simulink model "zhuangtaiguanceqi"  (R2022b)
settings: Solver=VariableStepAuto  StartTime=0.0  StopTime=100  RelTol=1e-3
settings Model: Creator=HONOR  LastModifiedBy=acer
settings DebuggingCC: UnconnectedInputMsg=warning  UnconnectedOutputMsg=warning  UnconnectedLineMsg=warning
settings ModelReferenceCC: EnableRefExpFcnMdlSchedulingChecks=on
settings RTWCC: DLArmComputeVersion=19.05

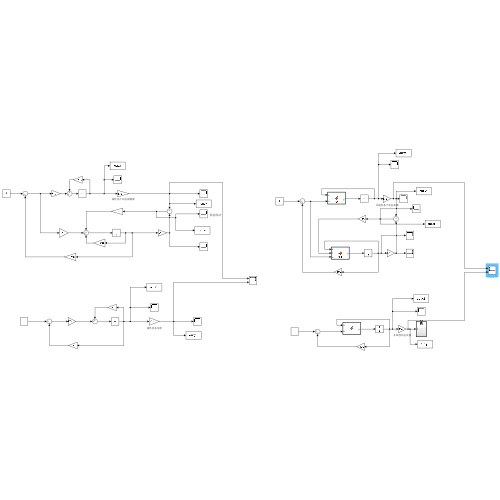
[thumbnail: Simulink's stored preview of the top-level diagram]
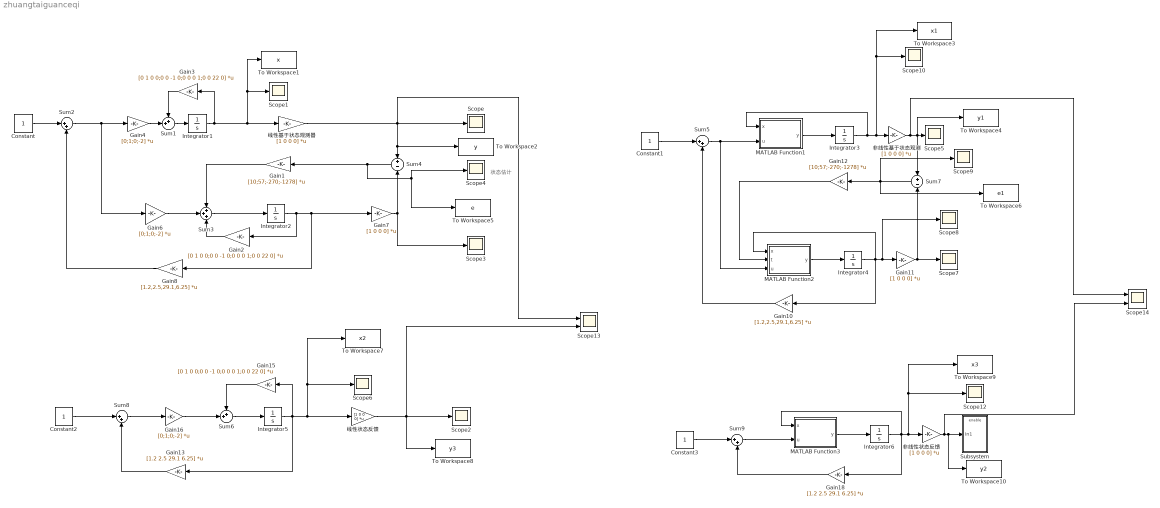
== system zhuangtaiguanceqi ==
  note: 状态估计
  Constant{,1..3} (4 alike) : Constant
  Gain1 : Gain  Gain=[10;57;-270;-1278]  Multiplication=Matrix(K*u)
  Gain10 : Gain  Gain=[1.2,2.5,29.1,6.25]  Multiplication=Matrix(K*u)
  Gain11 : Gain  Gain=[1 0 0 0]  Multiplication=Matrix(K*u)
  Gain12 : Gain  Gain=[10;57;-270;-1278]  Multiplication=Matrix(K*u)
  Gain13 : Gain  Gain=[1.2 2.5 29.1 6.25]  Multiplication=Matrix(K*u)
  Gain15 : Gain  Gain=[0 1 0 0;0 0 -1 0;0 0 0 1;0 0 22 0]  Multiplication=Matrix(K*u)
  Gain16 : Gain  Gain=[0;1;0;-2]  Multiplication=Matrix(K*u)
  Gain18 : Gain  Gain=[1.2 2.5 29.1 6.25]  Multiplication=Matrix(K*u)
  Gain2 : Gain  Gain=[0 1 0 0;0 0 -1 0;0 0 0 1;0 0 22 0]  Multiplication=Matrix(K*u)
  Gain3 : Gain  Gain=[0 1 0 0;0 0 -1 0;0 0 0 1;0 0 22 0]  Multiplication=Matrix(K*u)
  Gain4 : Gain  Gain=[0;1;0;-2]  Multiplication=Matrix(K*u)
  Gain6 : Gain  Gain=[0;1;0;-2]  Multiplication=Matrix(K*u)
  Gain7 : Gain  Gain=[1 0 0 0]  Multiplication=Matrix(K*u)
  Gain8 : Gain  Gain=[1.2,2.5,29.1,6.25]  Multiplication=Matrix(K*u)
  Integrator{1,3,5..6} (4 alike) : Integrator  InitialCondition=[0,0,0.1,0]
  Integrator2 : Integrator  InitialCondition=[0,0,0,0]
  Integrator4 : Integrator  InitialCondition=[0,0,0,0]
  MATLAB Function1 : MATLAB Function  TreatAsAtomicUnit=on
  MATLAB Function2 : MATLAB Function  TreatAsAtomicUnit=on
  MATLAB Function3 : MATLAB Function  TreatAsAtomicUnit=on
  Scope{,1..10,12} (12 alike) : Scope
  Scope13 : Scope  NumInputPorts=2
  Scope14 : Scope  NumInputPorts=2
  Subsystem : Subsystem
  Sum1 : Sum  Inputs=++|
  Sum{2,5,8..9} (4 alike) : Sum  Inputs=|++
  Sum3 : Sum  Inputs=+++
  Sum4 : Sum  Inputs=+-
  Sum6 : Sum  Inputs=++|
  Sum7 : Sum  Inputs=+-
  To Workspace1 : ToWorkspace  VariableName=x  SaveFormat=Structure With Time  SampleTime=-1
  To Workspace10 : ToWorkspace  VariableName=y2  SaveFormat=Structure With Time  SampleTime=-1
  To Workspace2 : ToWorkspace  VariableName=y  SaveFormat=Structure With Time  SampleTime=-1
  To Workspace3 : ToWorkspace  VariableName=x1  SaveFormat=Structure With Time  SampleTime=-1
  To Workspace4 : ToWorkspace  VariableName=y1  SaveFormat=Structure With Time  SampleTime=-1
  To Workspace5 : ToWorkspace  VariableName=e  SaveFormat=Structure With Time  SampleTime=-1
  To Workspace6 : ToWorkspace  VariableName=e1  SaveFormat=Structure With Time  SampleTime=-1
  To Workspace7 : ToWorkspace  VariableName=x2  SaveFormat=Structure With Time  SampleTime=-1
  To Workspace8 : ToWorkspace  VariableName=y3  SaveFormat=Structure With Time  SampleTime=-1
  To Workspace9 : ToWorkspace  VariableName=x3  SaveFormat=Structure With Time  SampleTime=-1
  线性基于状态观测器 : Gain  Gain=[1 0 0 0]  Multiplication=Matrix(K*u)
  线性状态反馈 : Gain  Gain=[1 0 0 0]  Multiplication=Matrix(K*u)
  非线性基于状态观测 : Gain  Gain=[1 0 0 0]  Multiplication=Matrix(K*u)
  非线性状态反馈 : Gain  Gain=[1 0 0 0]  Multiplication=Matrix(K*u)
  wires:
  Sum2/1 -> Gain6/1, Gain4/1
  Gain3/1 -> Sum1/1
  Integrator1/1 -> 线性基于状态观测器/1, To Workspace1/1, Scope1/1, Gain3/1
  Integrator2/1 -> Gain2/1, Gain8/1, Gain7/1
  线性基于状态观测器/1 -> Scope/1, Scope13/1, To Workspace2/1, Sum4/1
  Sum1/1 -> Integrator1/1
  Sum3/1 -> Integrator2/1
  Gain4/1 -> Sum1/2
  Sum4/1 -> Scope4/1, To Workspace5/1, Gain1/1
  Gain7/1 -> Scope3/1, Sum4/2
  Gain8/1 -> Sum2/2
  Constant/1 -> Sum2/1
  Sum5/1 -> MATLAB Function2/3(u), MATLAB Function1/2(u)
  Gain11/1 -> Sum7/2, Scope7/1
  MATLAB Function2/1(y) -> Integrator4/1
  Integrator4/1 -> Gain10/1, MATLAB Function2/1(x), Scope8/1, Gain11/1
  非线性基于状态观测/1 -> Scope14/1, To Workspace4/1, Sum7/1, Scope5/1
  Constant1/1 -> Sum5/1
  MATLAB Function1/1(y) -> Integrator3/1
  Integrator3/1 -> MATLAB Function1/1(x), Scope10/1, To Workspace3/1, 非线性基于状态观测/1
  Gain12/1 -> MATLAB Function2/2(t)
  Gain10/1 -> Sum5/2
  Sum7/1 -> Gain12/1, To Workspace6/1, Scope9/1
  Gain6/1 -> Sum3/2
  Gain2/1 -> Sum3/3
  Gain1/1 -> Sum3/1
  Sum9/1 -> MATLAB Function3/2(u)
  Constant2/1 -> Sum8/1
  Sum6/1 -> Integrator5/1
  Gain13/1 -> Sum8/2
  非线性状态反馈/1 -> Scope14/2, Subsystem/1(In1), To Workspace10/1
  Constant3/1 -> Sum9/1
  Sum8/1 -> Gain16/1
  MATLAB Function3/1(y) -> Integrator6/1
  Gain16/1 -> Sum6/2
  Gain15/1 -> Sum6/1
  Integrator6/1 -> Gain18/1, MATLAB Function3/1(x), To Workspace9/1, Scope12/1, 非线性状态反馈/1
  Gain18/1 -> Sum9/2
  Integrator5/1 -> 线性状态反馈/1, To Workspace7/1, Scope6/1, Gain15/1, Gain13/1
  线性状态反馈/1 -> Scope2/1, Scope13/2, To Workspace8/1

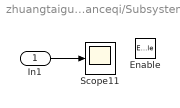
== system zhuangtaiguanceqi/Subsystem ==
  In1 : Inport
  Enable : EnablePort
  Scope11 : Scope
  wires:
  In1/1 -> Scope11/1

== matlab function zhuangtaiguanceqi/MATLAB Function2 ==
  data: x input; t input; u input; y output
function y = fcn(x, t, u)
M=1;
m=0.1;
l=0.5;
g=10;
Dx3=x(4)+t(3);
Dx4=(u*cos(x(3))-(M+m)*g*sin(x(3))+m*l*sin(x(3))*cos(x(3)*x(4)))/(m*l*cos(x(3))*cos(x(3))-(M+m)*l)+t(4);
Dx1=x(2)+t(1);
Dx2=((u+m*l*sin(x(3)*x(4)*x(4))-m*g*cos(x(3))*sin(x(3)))/(M+m-m*cos(x(3))*cos(x(3))))+t(2);
y=[Dx1;Dx2;Dx3;Dx4];

== matlab function zhuangtaiguanceqi/MATLAB Function3 ==
  data: x input; u input; y output
function y = fcn(x, u)
M=1;
m=0.1;
l=0.5;
g=10;
Dx3=x(4);
Dx4=(u*cos(x(3))-(M+m)*g*sin(x(3))+m*l*sin(x(3))*cos(x(3)*x(4)))/(m*l*cos(x(3))*cos(x(3))-(M+m)*l);
Dx1=x(2);
Dx2=((u+m*l*sin(x(3)*x(4)*x(4))-m*g*cos(x(3))*sin(x(3)))/(M+m-m*cos(x(3))*cos(x(3))));
y=[Dx1;Dx2;Dx3;Dx4];

== matlab function zhuangtaiguanceqi/MATLAB Function1 ==
  data: x input; u input; y output
function y = fcn(x, u)
M=1;
m=0.1;
l=0.5;
g=10;
Dx3=x(4);
Dx4=(u*cos(x(3))-(M+m)*g*sin(x(3))+m*l*sin(x(3))*cos(x(3)*x(4)))/(m*l*cos(x(3))*cos(x(3))-(M+m)*l);
Dx1=x(2);
Dx2=((u+m*l*sin(x(3)*x(4)*x(4))-m*g*cos(x(3))*sin(x(3)))/(M+m-m*cos(x(3))*cos(x(3))));
y=[Dx1;Dx2;Dx3;Dx4];
